simulink model "x7_2Simulink1"  (R2024b)
settings: Solver=VariableStepAuto  StartTime=0.0  StopTime=10.0  RelTol=1e-3
libraries: simulink x1, dspobslib x1
settings Model: Creator=Cory  LastModifiedBy=ryandavis
settings RTWCC: GPUComputeCapability=3.5

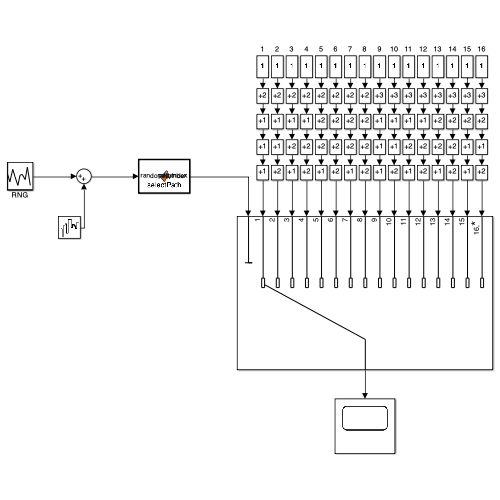
[thumbnail: Simulink's stored preview of the top-level diagram]
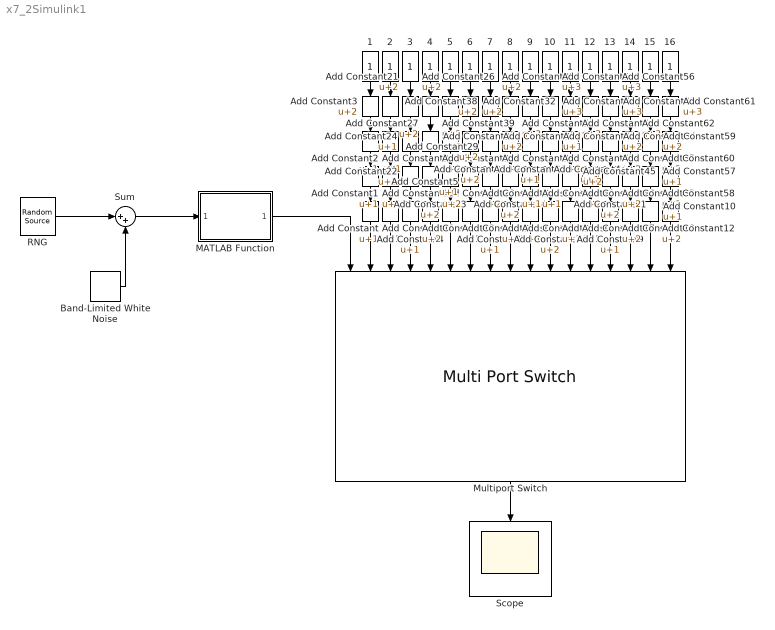
== system x7_2Simulink1 ==
  {1..16} (16 alike) : Constant
  Add Constant{,1..2,4..10,19..20,24..25,40..43,47..48,57..58} (22 alike) : Bias  Bias=1  SaturateOnIntegerOverflow=off
  Add Constant{3,11..18,21..23,26..39,45..46,51..52,54..55,59..60} (34 alike) : Bias  Bias=2  SaturateOnIntegerOverflow=off
  Add Constant{44,49..50,53,56,61..63} (8 alike) : Bias  Bias=3  SaturateOnIntegerOverflow=off
  Band-Limited White Noise : simulink/Sources/Band-Limited White Noise  Cov=[0.1]  Ts=0.1  seed=[23341]
  MATLAB Function : MATLAB Function  TreatAsAtomicUnit=on
  Multiport Switch : MultiPortSwitch  Inputs=16  OutMin=6  OutMax=10  OutDataTypeStr=double  SaturateOnIntegerOverflow=off  InputSameDT=off
  RNG : dspobslib/Random Source  SrcType=Gaussian  NormMethod=Ziggurat  CltLength=12  MinVal=0  MaxVal=1  MeanVal=0  VarVal=1  RepMode=Not repeatable  rawSeed=1  IsInherit=off  SampMode=Discrete  SampTime=10  SampFrame=1  DataType=Double  OutComplex=Real  OutputFrames=off
  Scope : Scope
  Sum : Sum  Inputs=|++
  wires:
  Add Constant/1 -> Multiport Switch/2
  Add Constant4/1 -> Multiport Switch/4
  Add Constant5/1 -> Multiport Switch/6
  Add Constant6/1 -> Multiport Switch/8
  Add Constant7/1 -> Multiport Switch/10
  Add Constant10/1 -> Multiport Switch/16
  Add Constant9/1 -> Multiport Switch/14
  Add Constant8/1 -> Multiport Switch/12
  Add Constant13/1 -> Multiport Switch/5
  Add Constant11/1 -> Multiport Switch/3
  Add Constant14/1 -> Multiport Switch/7
  Add Constant15/1 -> Multiport Switch/9
  Add Constant16/1 -> Multiport Switch/11
  Add Constant17/1 -> Multiport Switch/13
  Add Constant18/1 -> Multiport Switch/15
  Add Constant12/1 -> Multiport Switch/17
  Add Constant1/1 -> Add Constant/1
  Add Constant2/1 -> Add Constant1/1
  Add Constant3/1 -> Add Constant2/1
  1/1 -> Add Constant3/1
  Add Constant21/1 -> Add Constant20/1
  Add Constant20/1 -> Add Constant19/1
  2/1 -> Add Constant21/1
  Add Constant19/1 -> Add Constant11/1
  Add Constant26/1 -> Add Constant25/1
  4/1 -> Add Constant26/1
  Add Constant27/1 -> Add Constant24/1
  Add Constant24/1 -> Add Constant22/1
  Add Constant25/1 -> Add Constant23/1
  3/1 -> Add Constant27/1
  Add Constant23/1 -> Add Constant13/1
  Add Constant22/1 -> Add Constant4/1
  Add Constant32/1 -> Add Constant31/1
  6/1 -> Add Constant32/1
  Add Constant31/1 -> Add Constant29/1
  Add Constant39/1 -> Add Constant30/1
  Add Constant30/1 -> Add Constant28/1
  Add Constant35/1 -> Add Constant33/1
  Add Constant37/1 -> Add Constant36/1
  7/1 -> Add Constant38/1
  Add Constant36/1 -> Add Constant34/1
  5/1 -> Add Constant39/1
  8/1 -> Add Constant37/1
  Add Constant38/1 -> Add Constant35/1
  Add Constant28/1 -> Add Constant5/1
  Add Constant29/1 -> Add Constant14/1
  Add Constant34/1 -> Add Constant15/1
  Add Constant33/1 -> Add Constant6/1
  Add Constant44/1 -> Add Constant43/1
  10/1 -> Add Constant44/1
  Add Constant43/1 -> Add Constant41/1
  Add Constant53/1 -> Add Constant42/1
  Add Constant60/1 -> Add Constant58/1
  Add Constant55/1 -> Add Constant52/1
  Add Constant63/1 -> Add Constant54/1
  13/1 -> Add Constant63/1
  Add Constant61/1 -> Add Constant60/1
  Add Constant59/1 -> Add Constant57/1
  15/1 -> Add Constant62/1
  Add Constant54/1 -> Add Constant51/1
  Add Constant42/1 -> Add Constant40/1
  Add Constant47/1 -> Add Constant45/1
  Add Constant56/1 -> Add Constant55/1
  Add Constant49/1 -> Add Constant48/1
  11/1 -> Add Constant50/1
  14/1 -> Add Constant56/1
  Add Constant48/1 -> Add Constant46/1
  16/1 -> Add Constant61/1
  9/1 -> Add Constant53/1
  12/1 -> Add Constant49/1
  Add Constant50/1 -> Add Constant47/1
  Add Constant62/1 -> Add Constant59/1
  Add Constant58/1 -> Add Constant12/1
  Add Constant57/1 -> Add Constant10/1
  Add Constant52/1 -> Add Constant18/1
  Add Constant51/1 -> Add Constant9/1
  Add Constant46/1 -> Add Constant17/1
  Add Constant45/1 -> Add Constant8/1
  Add Constant41/1 -> Add Constant16/1
  Add Constant40/1 -> Add Constant7/1
  MATLAB Function/1(pathIndex) -> Multiport Switch/1
  Multiport Switch/1 -> Scope/1
  RNG/1 -> Sum/1
  Band-Limited White Noise/1 -> Sum/2
  Sum/1 -> MATLAB Function/1(randomNumber)

== matlab function x7_2Simulink1/MATLAB Function ==
  data: randomNumber input; pathIndex output
function pathIndex = selectPath(randomNumber) %#codegen
    % Clamp the random number to stay within [0, 1]
    randomNumber = max(0, min(randomNumber, 1));
    
    % Initialize pathIndex to zero (or any valid default value)
    pathIndex = int32(0);

    % Check the value of randomNumber and assign pathIndex accordingly
    if randomNumber >= 0 && randomNumber <= 0.0252
        pathIndex = int32(1);  % Path 1
    elseif randomNumber > 0.0252 && randomNumber <= 0.0840
        pathIndex = int32(2);  % Path 2
    elseif randomNumber > 0.0840 && randomNumber <= 0.0984
        pathIndex = int32(3);  % Path 3
    elseif randomNumber > 0.0984 && randomNumber <= 0.1200
        pathIndex = int32(4);  % Path 4
    elseif randomNumber > 0.1200 && randomNumber <= 0.1620
        pathIndex = int32(5);  % Path 5
    elseif randomNumber > 0.1620 && randomNumber <= 0.2040
        pathIndex = int32(6);  % Path 6
    elseif randomNumber > 0.2040 && randomNumber <= 0.2628
        pathIndex = int32(7);  % Path 7
    elseif randomNumber > 0.2628 && randomNumber <= 0.4000
        pathIndex = int32(8);  % Path 8
    elseif randomNumber > 0.4000 && randomNumber <= 0.5200
        pathIndex = int32(9);  % Path 9
    elseif randomNumber > 0.5200 && randomNumber <= 0.6400
        pathIndex = int32(10); % Path 10
    elseif randomNumber > 0.6400 && randomNumber <= 0.6760
        pathIndex = int32(11); % Path 11
    elseif randomNumber > 0.6760 && randomNumber <= 0.7000
        pathIndex = int32(12); % Path 12
    elseif randomNumber > 0.7000 && randomNumber <= 0.7450
        pathIndex = int32(13); % Path 13
    elseif randomNumber > 0.7450 && randomNumber <= 0.8500
        pathIndex = int32(14); % Path 14
    elseif randomNumber > 0.8500 && randomNumber <= 0.9250
        pathIndex = int32(15); % Path 15
    elseif randomNumber > 0.9250 && randomNumber <= 1.0000
        pathIndex = int32(16); % Path 16
    end

    % Optional: Add a warning if pathIndex remains 0
    if pathIndex == int32(0)
        warning('randomNumber is out of expected range: %f', randomNumber);
    end
end
